simulink model "euler321_I2B_12B_tmp"  (Simulink 9.0)
settings: Solver=ode3  StartTime=0.0  StopTime=10.0  FixedStep=0.01  RelTol=1e-3  EnableMultiTasking=on
settings Model: Creator=elliocm  LastModifiedBy=hbourbou
settings DataIOCC: LimitDataPoints=on  SaveFormat=StructureWithTime  SignalLoggingSaveFormat=ModelDataLogs
settings OptimizationCC: ExpressionDepthLimit=2147483647
settings DebuggingCC: SolverPrmCheckMsg=warning  FcnCallInpInsideContextMsg=warning  StateNameClashWarn=warning
settings GRTTargetCC: GeneratePreprocessorConditionals=Disable all  CombineOutputUpdateFcns=off  GRTInterface=on

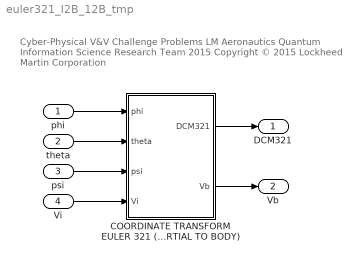
== system euler321_I2B_12B_tmp ==
  note: Cyber-Physical V&V Challenge Problems
      | LM Aeronautics Quantum Information Science Research Team 2015
      | Copyright © 2015 Lockheed Martin Corporation
  phi : Inport  OutDataTypeStr=double
  theta : Inport  Port=2  OutDataTypeStr=double
  psi : Inport  Port=3  OutDataTypeStr=double
  Vi : Inport  Port=4  OutDataTypeStr=double  PortDimensions=3
  COORDINATE TRANSFORM EULER 321 (INERTIAL TO BODY) : Subsystem
  DCM321 : Outport  VectorParamsAs1DForOutWhenUnconnected=off
  Vb : Outport  Port=2  VectorParamsAs1DForOutWhenUnconnected=off
  wires:
  COORDINATE TRANSFORM EULER 321 (INERTIAL TO BODY)/1(DCM321) -> DCM321/1
  COORDINATE TRANSFORM EULER 321 (INERTIAL TO BODY)/2(Vb) -> Vb/1
  phi/1 -> COORDINATE TRANSFORM EULER 321 (INERTIAL TO BODY)/1(phi)
  theta/1 -> COORDINATE TRANSFORM EULER 321 (INERTIAL TO BODY)/2(theta)
  psi/1 -> COORDINATE TRANSFORM EULER 321 (INERTIAL TO BODY)/3(psi)
  Vi/1 -> COORDINATE TRANSFORM EULER 321 (INERTIAL TO BODY)/4(Vi)

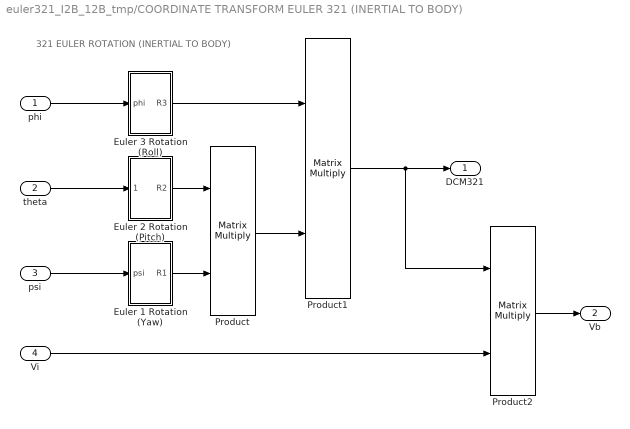
== system euler321_I2B_12B_tmp/COORDINATE TRANSFORM EULER 321 (INERTIAL TO BODY) ==
  note: 321 EULER ROTATION (INERTIAL TO BODY)
  phi : Inport
  theta : Inport  Port=2
  psi : Inport  Port=3
  Vi : Inport  Port=4
  Euler 1 Rotation (Yaw) : Subsystem
  Euler 2 Rotation (Pitch) : Subsystem
  Euler 3 Rotation (Roll) : Subsystem
  Product : Product  Multiplication=Matrix(*)  RndMeth=Zero
  Product1 : Product  Multiplication=Matrix(*)  RndMeth=Zero
  Product2 : Product  Multiplication=Matrix(*)  RndMeth=Zero
  DCM321 : Outport  VectorParamsAs1DForOutWhenUnconnected=off
  Vb : Outport  Port=2  VectorParamsAs1DForOutWhenUnconnected=off
  wires:
  Euler 2 Rotation (Pitch)/1(R2) -> Product/1
  Euler 1 Rotation (Yaw)/1(R1) -> Product/2
  Euler 3 Rotation (Roll)/1(R3) -> Product1/1
  Product/1 -> Product1/2
  Product1/1 -> DCM321/1, Product2/1
  Product2/1 -> Vb/1
  phi/1 -> Euler 3 Rotation (Roll)/1(phi)
  theta/1 -> Euler 2 Rotation (Pitch)/1(theta)
  psi/1 -> Euler 1 Rotation (Yaw)/1(psi)
  Vi/1 -> Product2/2

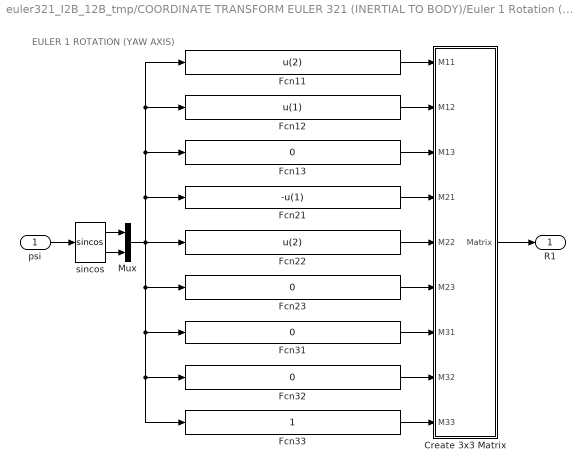
== system euler321_I2B_12B_tmp/COORDINATE TRANSFORM EULER 321 (INERTIAL TO BODY)/Euler 1 Rotation (Yaw) ==
  note: EULER 1 ROTATION (YAW AXIS)
  psi : Inport
  Create 3x3 Matrix : Subsystem  mask(Create 3x3 Matrix){}
      mask help: shared_aeroblks:sharedaeroblkutil:blockCreate3x3MatrixDesc
      mask init:
      | if license('test','aerospace_blockset')
      |     aerosharedicon('shared');
      | elseif license('test','powertrain_blockset')
      |     sharedautoicon('shared');
      | end
      mask Help: eval('if license(''test'',''aerospace_blockset'')aerosharedhelp(''create_threebythree_matrix'');elseif license(''test'',''powertrain_blockset'')sharedautohelp(''create_threebythree_matrix'');end')
      mask Display:
      | port_label('input',1,'A_{11}','texmode','on');
      | port_label('input',2,'A_{12}','texmode','on');
      | port_label('input',3,'A_{13}','texmode','on');
      | port_label('input',4,'A_{21}','texmode','on');
      | port_label('input',5,'A_{22}','texmode','on');
      | port_label('input',6,'A_{23}','texmode','on');
      | port_label('input',7,'A_{31}','texmode','on');
      | port_label('input',8,'A_{32}','texmode','on');
      | port_label('input',9,'A_{33}','texmode','on');
      | port_label('output',1,'A','texmode','on');
  Fcn11 : Fcn  Expr=u(2)
  Fcn12 : Fcn  Expr=u(1)
  Fcn{13,23,31..32} (4 alike) : Fcn  Expr=0
  Fcn21 : Fcn  Expr=-u(1)
  Fcn22 : Fcn  Expr=u(2)
  Fcn33 : Fcn  Expr=1
  Mux : Mux  Inputs=2
  sincos : Trigonometry  Operator=sincos
  R1 : Outport  PortDimensions=[3,3]  VectorParamsAs1DForOutWhenUnconnected=off
  wires:
  psi/1 -> sincos/1
  Create 3x3 Matrix/1(Matrix) -> R1/1
  sincos/1 -> Mux/1
  sincos/2 -> Mux/2
  Mux/1 -> Fcn32/1, Fcn33/1, Fcn31/1, Fcn23/1, Fcn22/1, Fcn11/1, Fcn12/1, Fcn13/1, Fcn21/1
  Fcn11/1 -> Create 3x3 Matrix/1(M11)
  Fcn12/1 -> Create 3x3 Matrix/2(M12)
  Fcn13/1 -> Create 3x3 Matrix/3(M13)
  Fcn21/1 -> Create 3x3 Matrix/4(M21)
  Fcn31/1 -> Create 3x3 Matrix/7(M31)
  Fcn22/1 -> Create 3x3 Matrix/5(M22)
  Fcn23/1 -> Create 3x3 Matrix/6(M23)
  Fcn32/1 -> Create 3x3 Matrix/8(M32)
  Fcn33/1 -> Create 3x3 Matrix/9(M33)

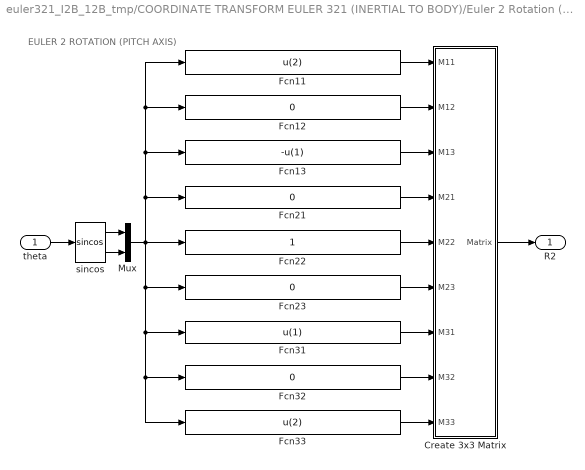
== system euler321_I2B_12B_tmp/COORDINATE TRANSFORM EULER 321 (INERTIAL TO BODY)/Euler 2 Rotation (Pitch) ==
  note: EULER 2 ROTATION (PITCH AXIS)
  theta : Inport
  Create 3x3 Matrix : Subsystem  mask(Create 3x3 Matrix){}
      mask help: shared_aeroblks:sharedaeroblkutil:blockCreate3x3MatrixDesc
      mask init:
      | if license('test','aerospace_blockset')
      |     aerosharedicon('shared');
      | elseif license('test','powertrain_blockset')
      |     sharedautoicon('shared');
      | end
      mask Help: eval('if license(''test'',''aerospace_blockset'')aerosharedhelp(''create_threebythree_matrix'');elseif license(''test'',''powertrain_blockset'')sharedautohelp(''create_threebythree_matrix'');end')
      mask Display:
      | port_label('input',1,'A_{11}','texmode','on');
      | port_label('input',2,'A_{12}','texmode','on');
      | port_label('input',3,'A_{13}','texmode','on');
      | port_label('input',4,'A_{21}','texmode','on');
      | port_label('input',5,'A_{22}','texmode','on');
      | port_label('input',6,'A_{23}','texmode','on');
      | port_label('input',7,'A_{31}','texmode','on');
      | port_label('input',8,'A_{32}','texmode','on');
      | port_label('input',9,'A_{33}','texmode','on');
      | port_label('output',1,'A','texmode','on');
  Fcn11 : Fcn  Expr=u(2)
  Fcn{12,21,23,32} (4 alike) : Fcn  Expr=0
  Fcn13 : Fcn  Expr=-u(1)
  Fcn22 : Fcn  Expr=1
  Fcn31 : Fcn  Expr=u(1)
  Fcn33 : Fcn  Expr=u(2)
  Mux : Mux  Inputs=2
  sincos : Trigonometry  Operator=sincos
  R2 : Outport  PortDimensions=[3,3]  VectorParamsAs1DForOutWhenUnconnected=off
  wires:
  theta/1 -> sincos/1
  Create 3x3 Matrix/1(Matrix) -> R2/1
  sincos/1 -> Mux/1
  sincos/2 -> Mux/2
  Mux/1 -> Fcn32/1, Fcn33/1, Fcn31/1, Fcn23/1, Fcn22/1, Fcn11/1, Fcn12/1, Fcn13/1, Fcn21/1
  Fcn11/1 -> Create 3x3 Matrix/1(M11)
  Fcn12/1 -> Create 3x3 Matrix/2(M12)
  Fcn13/1 -> Create 3x3 Matrix/3(M13)
  Fcn21/1 -> Create 3x3 Matrix/4(M21)
  Fcn31/1 -> Create 3x3 Matrix/7(M31)
  Fcn22/1 -> Create 3x3 Matrix/5(M22)
  Fcn23/1 -> Create 3x3 Matrix/6(M23)
  Fcn32/1 -> Create 3x3 Matrix/8(M32)
  Fcn33/1 -> Create 3x3 Matrix/9(M33)

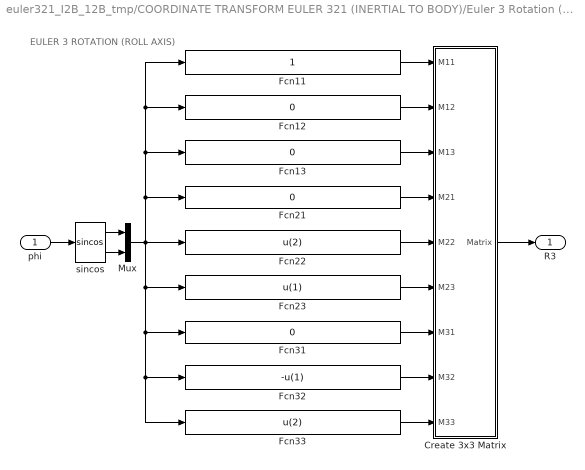
== system euler321_I2B_12B_tmp/COORDINATE TRANSFORM EULER 321 (INERTIAL TO BODY)/Euler 3 Rotation (Roll) ==
  note: EULER 3 ROTATION (ROLL AXIS)
  phi : Inport
  Create 3x3 Matrix : Subsystem  mask(Create 3x3 Matrix){}
      mask help: shared_aeroblks:sharedaeroblkutil:blockCreate3x3MatrixDesc
      mask init:
      | if license('test','aerospace_blockset')
      |     aerosharedicon('shared');
      | elseif license('test','powertrain_blockset')
      |     sharedautoicon('shared');
      | end
      mask Help: eval('if license(''test'',''aerospace_blockset'')aerosharedhelp(''create_threebythree_matrix'');elseif license(''test'',''powertrain_blockset'')sharedautohelp(''create_threebythree_matrix'');end')
      mask Display:
      | port_label('input',1,'A_{11}','texmode','on');
      | port_label('input',2,'A_{12}','texmode','on');
      | port_label('input',3,'A_{13}','texmode','on');
      | port_label('input',4,'A_{21}','texmode','on');
      | port_label('input',5,'A_{22}','texmode','on');
      | port_label('input',6,'A_{23}','texmode','on');
      | port_label('input',7,'A_{31}','texmode','on');
      | port_label('input',8,'A_{32}','texmode','on');
      | port_label('input',9,'A_{33}','texmode','on');
      | port_label('output',1,'A','texmode','on');
  Fcn11 : Fcn  Expr=1
  Fcn{12..13,21,31} (4 alike) : Fcn  Expr=0
  Fcn22 : Fcn  Expr=u(2)
  Fcn23 : Fcn  Expr=u(1)
  Fcn32 : Fcn  Expr=-u(1)
  Fcn33 : Fcn  Expr=u(2)
  Mux : Mux  Inputs=2
  sincos : Trigonometry  Operator=sincos
  R3 : Outport  PortDimensions=[3,3]  VectorParamsAs1DForOutWhenUnconnected=off
  wires:
  phi/1 -> sincos/1
  Create 3x3 Matrix/1(Matrix) -> R3/1
  sincos/1 -> Mux/1
  sincos/2 -> Mux/2
  Mux/1 -> Fcn32/1, Fcn33/1, Fcn31/1, Fcn23/1, Fcn22/1, Fcn11/1, Fcn12/1, Fcn13/1, Fcn21/1
  Fcn11/1 -> Create 3x3 Matrix/1(M11)
  Fcn12/1 -> Create 3x3 Matrix/2(M12)
  Fcn13/1 -> Create 3x3 Matrix/3(M13)
  Fcn21/1 -> Create 3x3 Matrix/4(M21)
  Fcn31/1 -> Create 3x3 Matrix/7(M31)
  Fcn22/1 -> Create 3x3 Matrix/5(M22)
  Fcn23/1 -> Create 3x3 Matrix/6(M23)
  Fcn32/1 -> Create 3x3 Matrix/8(M32)
  Fcn33/1 -> Create 3x3 Matrix/9(M33)

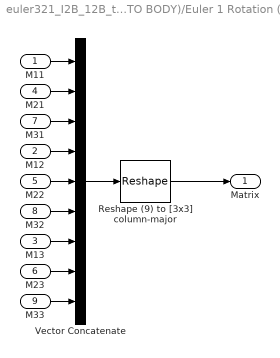
== system euler321_I2B_12B_tmp/COORDINATE TRANSFORM EULER 321 (INERTIAL TO BODY)/Euler 1 Rotation (Yaw)/Create 3x3 Matrix ==
  M11 : Inport  PortDimensions=1
  M12 : Inport  Port=2  PortDimensions=1
  M13 : Inport  Port=3  PortDimensions=1
  M21 : Inport  Port=4  PortDimensions=1
  M22 : Inport  Port=5  PortDimensions=1
  M23 : Inport  Port=6  PortDimensions=1
  M31 : Inport  Port=7  PortDimensions=1
  M32 : Inport  Port=8  PortDimensions=1
  M33 : Inport  Port=9  PortDimensions=1
  Reshape (9) to [3x3] column-major : Reshape  OutputDimensionality=Customize  OutputDimensions=[3,3]
  Vector Concatenate : Concatenate  NumInputs=9
  Matrix : Outport  PortDimensions=[3 3]  VectorParamsAs1DForOutWhenUnconnected=off
  wires:
  M33/1 -> Vector Concatenate/9
  M23/1 -> Vector Concatenate/8
  M13/1 -> Vector Concatenate/7
  M32/1 -> Vector Concatenate/6
  Reshape (9) to [3x3] column-major/1 -> Matrix/1
  M22/1 -> Vector Concatenate/5
  M12/1 -> Vector Concatenate/4
  M31/1 -> Vector Concatenate/3
  M21/1 -> Vector Concatenate/2
  M11/1 -> Vector Concatenate/1
  Vector Concatenate/1 -> Reshape (9) to [3x3] column-major/1

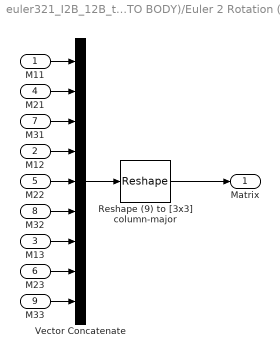
== system euler321_I2B_12B_tmp/COORDINATE TRANSFORM EULER 321 (INERTIAL TO BODY)/Euler 2 Rotation (Pitch)/Create 3x3 Matrix ==
  M11 : Inport  PortDimensions=1
  M12 : Inport  Port=2  PortDimensions=1
  M13 : Inport  Port=3  PortDimensions=1
  M21 : Inport  Port=4  PortDimensions=1
  M22 : Inport  Port=5  PortDimensions=1
  M23 : Inport  Port=6  PortDimensions=1
  M31 : Inport  Port=7  PortDimensions=1
  M32 : Inport  Port=8  PortDimensions=1
  M33 : Inport  Port=9  PortDimensions=1
  Reshape (9) to [3x3] column-major : Reshape  OutputDimensionality=Customize  OutputDimensions=[3,3]
  Vector Concatenate : Concatenate  NumInputs=9
  Matrix : Outport  PortDimensions=[3 3]  VectorParamsAs1DForOutWhenUnconnected=off
  wires:
  M33/1 -> Vector Concatenate/9
  M23/1 -> Vector Concatenate/8
  M13/1 -> Vector Concatenate/7
  M32/1 -> Vector Concatenate/6
  Reshape (9) to [3x3] column-major/1 -> Matrix/1
  M22/1 -> Vector Concatenate/5
  M12/1 -> Vector Concatenate/4
  M31/1 -> Vector Concatenate/3
  M21/1 -> Vector Concatenate/2
  M11/1 -> Vector Concatenate/1
  Vector Concatenate/1 -> Reshape (9) to [3x3] column-major/1

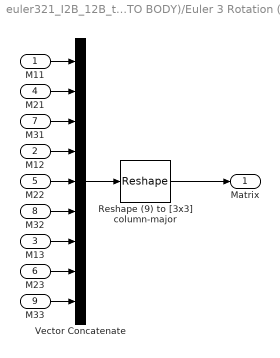
== system euler321_I2B_12B_tmp/COORDINATE TRANSFORM EULER 321 (INERTIAL TO BODY)/Euler 3 Rotation (Roll)/Create 3x3 Matrix ==
  M11 : Inport  PortDimensions=1
  M12 : Inport  Port=2  PortDimensions=1
  M13 : Inport  Port=3  PortDimensions=1
  M21 : Inport  Port=4  PortDimensions=1
  M22 : Inport  Port=5  PortDimensions=1
  M23 : Inport  Port=6  PortDimensions=1
  M31 : Inport  Port=7  PortDimensions=1
  M32 : Inport  Port=8  PortDimensions=1
  M33 : Inport  Port=9  PortDimensions=1
  Reshape (9) to [3x3] column-major : Reshape  OutputDimensionality=Customize  OutputDimensions=[3,3]
  Vector Concatenate : Concatenate  NumInputs=9
  Matrix : Outport  PortDimensions=[3 3]  VectorParamsAs1DForOutWhenUnconnected=off
  wires:
  M33/1 -> Vector Concatenate/9
  M23/1 -> Vector Concatenate/8
  M13/1 -> Vector Concatenate/7
  M32/1 -> Vector Concatenate/6
  Reshape (9) to [3x3] column-major/1 -> Matrix/1
  M22/1 -> Vector Concatenate/5
  M12/1 -> Vector Concatenate/4
  M31/1 -> Vector Concatenate/3
  M21/1 -> Vector Concatenate/2
  M11/1 -> Vector Concatenate/1
  Vector Concatenate/1 -> Reshape (9) to [3x3] column-major/1
